simulink model "ts_asf_two_a_2017a"  (R2017a)
settings: Solver=ode45  StartTime=0.0  StopTime=10  RelTol=1e-3  EnableMultiTasking=on
values from neighbouring files (symbols this model uses):
  A = plant_linear_A    [design_digital.m]
  B = plant_linear_B    [design_digital.m]
  C = [1 0 0 0 0 0;0 0 0 0 1 0]    [design_digital.m]
  K1 = Kd(:,1:6)    [design_digital.m]
  K2 = Kd(:,7:8)    [design_digital.m]
undefined symbols (not defined in the file or in its folder): Aa, Ba
libraries: simulink x2
settings Model: Creator=rjv  LastModifiedBy=kando
settings DataIOCC: LimitDataPoints=on  SaveFormat=Array
settings OptimizationCC: LifeSpan=inf
settings DebuggingCC: AllowSymbolicDim=off  SFUnexpectedBacktrackingDiag=warning  SFNoUnconditionalDefaultTransitionDiag=warning  SFExecutionAtInitializationDiag=none
settings HardwareCC: ProdBitPerPointer=32  ProdBitPerSizeT=32  ProdBitPerPtrDiffT=32  ProdLargestAtomicFloat=None  ProdIntDivRoundTo=Undefined  ProdEndianess=Unspecified  ProdWordSize=32  ProdHWDeviceType=32-bit Generic
settings ModelReferenceCC: PropagateSignalLabelsOutOfModel=off
settings GRTTargetCC: TargetLangStandard=C89/C90 (ANSI)  GeneratePreprocessorConditionals=Disable all
settings ConfigComp: CovMetricSettings=dw  CovHtmlReporting=on  CovSaveCumulativeToWorkspaceVar=on  CovSaveSingleToWorkspaceVar=on  CovExternalEMLEnable=off

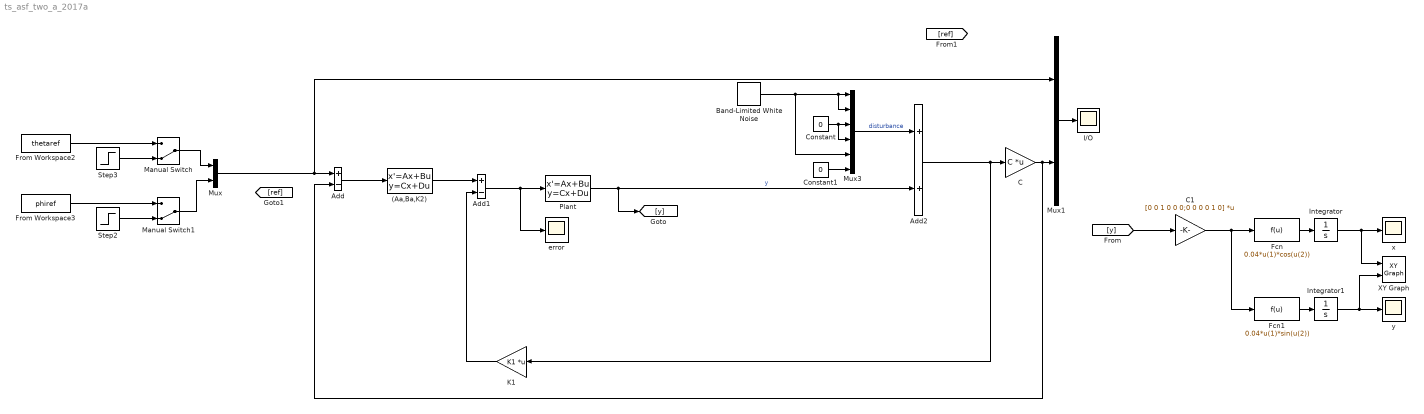
== system ts_asf_two_a_2017a ==
  (Aa,Ba,K2) : StateSpace  A=Aa  B=Ba  C=K2  D=0*K2*Ba  X0=K2\(K1*[0;0;0;0;pi/4;0])
  Add : Sum  Inputs=+-
  Add1 : Sum  Inputs=+-
  Add2 : Sum
  Band-Limited White Noise : simulink/Sources/Band-Limited White Noise  Cov=1e-8  Ts=0.01  seed=[23341]
  C : Gain  Gain=C  Multiplication=Matrix(K*u)
  C1 : Gain  Gain=[0 0 1 0 0 0;0 0 0 0 1 0]  Multiplication=Matrix(K*u)
  Constant : Constant  Value=0
  Constant1 : Constant  Value=0
  Fcn : Fcn  Expr=0.04*u(1)*cos(u(2))
  Fcn1 : Fcn  Expr=0.04*u(1)*sin(u(2))
  From Workspace2 : FromWorkspace  VariableName=thetaref  SampleTime=0.01  OutputAfterFinalValue=Holding final value
  From Workspace3 : FromWorkspace  VariableName=phiref  SampleTime=0.01  OutputAfterFinalValue=Holding final value
  I/O : Scope
  Integrator : Integrator
  Integrator1 : Integrator
  K1 : Gain  Gain=K1  Multiplication=Matrix(K*u)
  Manual Switch : ManualSwitch  CurrentSetting=0
  Manual Switch1 : ManualSwitch  CurrentSetting=0
  Mux : Mux  Inputs=2
  Mux1 : Mux  Inputs=2
  Mux3 : Mux  Inputs=6
  Plant : StateSpace  A=A  B=B  C=eye(length(A))  D=zeros(length(A),min(size((B))))  X0=[0;0;0;0;pi/4;0]
  Step2 : Step  Time=0  Before=pi/4  After=pi/4+1  SampleTime=0
  Step3 : Step  Time=0  After=5  SampleTime=0
  XY Graph : simulink/Sinks/XY Graph  xmin=-1  xmax=1  ymin=-1  ymax=1  st=-1
  error : Scope
  x : Scope
  y : Scope
  wires:
  Add1/1 -> error/1, Plant/1
  (Aa,Ba,K2)/1 -> Add1/1
  Add/1 -> (Aa,Ba,K2)/1
  K1/1 -> Add1/2
  C/1 -> Add/2, Mux1/2
  Fcn/1 -> Integrator/1
  Fcn1/1 -> Integrator1/1
  Integrator/1 -> x/1, XY Graph/1
  Integrator1/1 -> XY Graph/2, y/1
  C1/1 -> Fcn/1, Fcn1/1
  Mux1/1 -> I/O/1
  Mux/1 -> Mux1/1, Add/1
  Add2/1 -> K1/1, C/1
  Mux3/1 -> Add2/1  "disturbance"
  Band-Limited White Noise/1 -> Mux3/5, Mux3/2, Mux3/1
  Constant/1 -> Mux3/4, Mux3/3
  Plant/1 -> [y], Add2/2  "y"
  Step2/1 -> Manual Switch1/2
  From Workspace3/1 -> Manual Switch1/1
  Manual Switch1/1 -> Mux/2
  Manual Switch/1 -> Mux/1
  Step3/1 -> Manual Switch/2
  From Workspace2/1 -> Manual Switch/1
  Constant1/1 -> Mux3/6
  [y] -> C1/1
